simulink library "ifo"  (Simulink 8.2)
settings: Solver=ode45  StartTime=0.0  StopTime=10.0  RelTol=1e-3
undefined symbols (not defined in the file or in its folder): ENUM_EPSADASABREASON_NO_DRIVING_INTERRUPTION, ENUM_GEARPOSN_1ST, ENUM_GEARPOSN_2ND, ENUM_GEARPOSN_3RD, ENUM_GEARPOSN_4TH, ENUM_GEARPOSN_5TH, ENUM_GEARPOSN_6TH, ENUM_LFCSTATE_AUTOSTEERING, ENUM_LFCSTATE_DEGRADED, ENUM_SHIFTLEVER_D, ENUM_SHIFTLEVER_D2, ENUM_SHIFTLEVER_D3, FALSE, KAPP_VehicleWidth_m, KIFO_C1Max4Act_rad, KIFO_C2Max4Act_rat, KIFO_C2Max4Disable_rat, KIFO_C2Max4DisableThr_s, KIFO_DriverStrFightConfirmTime_s, KIFO_DriverStrFightResetTime_s, KIFO_DriverStrFightSetTime_s, KIFO_DriverStrFightThres_Nm, KIFO_DriverStrFightThresHys_Nm, KIFO_DriverStrSoftConfirmTime_s, KIFO_DriverStrSoftResetTime_s, KIFO_DriverStrSoftSetTime_s, KIFO_DriverStrSoftThres_Nm, KIFO_DriverStrStrongConfirmTime_s, KIFO_DriverStrStrongResetTime_s, KIFO_DriverStrStrongSetTime_s, KIFO_DriverStrStrongThres_Nm, KIFO_DriverStrStrongThresHys_Nm, KIFO_Lane4ActThr_s, KIFO_LaneWidthLowThr_m, KIFO_LaneWidthUpThr_m, KIFO_LFCVehSpdMaxLimition_kph, KIFO_LFCVehSpdMimLimition_kph, KIFO_LKAMaxActSpeed_kph, KIFO_LKAMaxDeactSpeed_kph, KIFO_LKAMinActSpeed_kph, KIFO_LKAMinDeactSpeed_kph, KIFO_TLCTriggerThrHysis_s, KIFO_TurnSignalSwOFFTime_s, MIFO_TLCThr4LKA_s, TRUE
libraries: hcu_lib x41, simulink x11, hmi x1, gaps x1, ttc x1, sft x1, veh x1
(part 2 of 2)

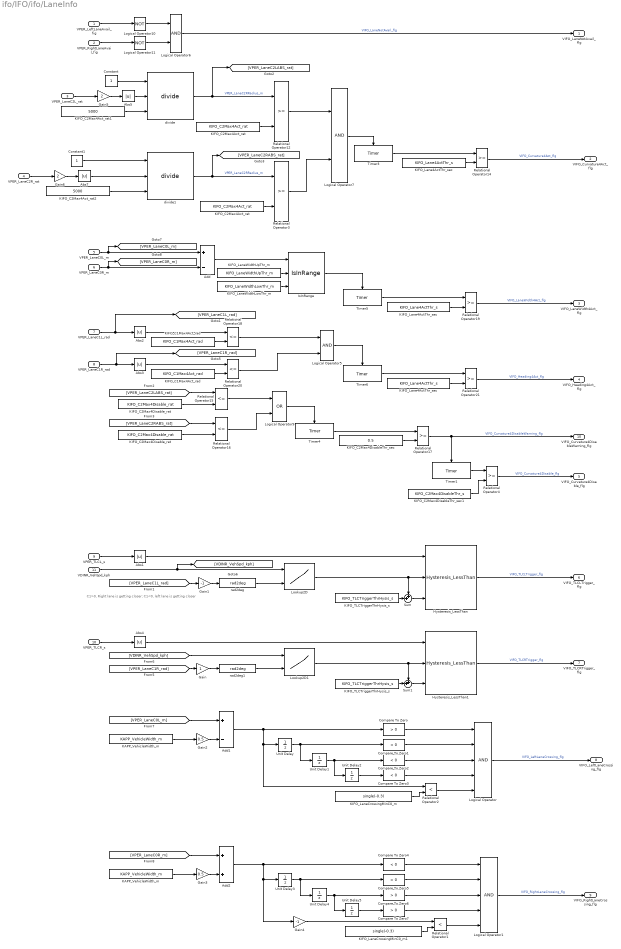
== system ifo/IFO/ifo/LaneInfo ==
  note: C1>0, Right lane is getting closer; C1<0, left lane is getting closer
  "VPER_LeftLaneAvail_fig " : Inport
  "VPER_RightLaneAvail_fig " : Inport  Port=2
  VPER_LaneC2L_rat : Inport  Port=3
  VPER_LaneC2R_rat : Inport  Port=4
  VPER_LaneC0L_m : Inport  Port=5
  VPER_LaneC0R_m : Inport  Port=6
  VPER_LaneC1L_rad : Inport  Port=7
  VPER_LaneC1R_rad : Inport  Port=8
  VPER_TLCL_s : Inport  Port=9
  VPER_TLCR_s : Inport  Port=10
  VDINR_VehSpd_kph : Inport  Port=11
  Abs{1..5,7} (6 alike) : Abs
  Add : Sum  Inputs=+-
  Add1 : Sum  Inputs=+-
  Add2 : Sum
  Compare To Zero{,5..7} (4 alike) : simulink/Logic and Bit Operations/Compare To Zero  relop=>  OutDataTypeStr=boolean
  Compare To Zero{1..4} (4 alike) : simulink/Logic and Bit Operations/Compare To Zero  relop=<  OutDataTypeStr=boolean
  Constant : Constant  OutDataTypeStr=single
  Constant1 : Constant  OutDataTypeStr=single
  Gain : Gain
  Gain1 : Gain  Gain=-1
  Gain2 : Gain  Gain=0.5
  Gain3 : Gain  Gain=0.5
  Gain4 : Gain  Gain=-1
  Gain5 : Gain  Gain=2
  Gain6 : Gain  Gain=2
  Hysteresis_LessThan : hcu_lib/Hysteresis_LessThan  SystemSampleTime=-1
  Hysteresis_LessThan1 : hcu_lib/Hysteresis_LessThan  SystemSampleTime=-1
  IsInRange : hcu_lib/IsInRange  SystemSampleTime=-1
  KAPP_VehicleWidth_m : Constant  Value=KAPP_VehicleWidth_m
  "KAPP_VehicleWidth_m " : Constant  Value=KAPP_VehicleWidth_m
  KIFO_C1Max4Act_rad : Constant  Value=KIFO_C1Max4Act_rad
  "KIFO_C1Max4Act_rad " : Constant  Value=KIFO_C1Max4Act_rad
  KIFO_C2Max4Act_rat : Constant  Value=KIFO_C2Max4Act_rat
  "KIFO_C2Max4Act_rat " : Constant  Value=KIFO_C2Max4Act_rat
  KIFO_C2Max4Act_rat1 : Constant  Value=5000  OutDataTypeStr=single
  KIFO_C2Max4Act_rat2 : Constant  Value=5000  OutDataTypeStr=single
  KIFO_C2Max4DisableThr_sec : Constant  Value=0.5
  KIFO_C2Max4DisableThr_sec1 : Constant  Value=KIFO_C2Max4DisableThr_s
  KIFO_C2Max4Disable_rat : Constant  Value=KIFO_C2Max4Disable_rat
  "KIFO_C2Max4Disable_rat " : Constant  Value=KIFO_C2Max4Disable_rat
  KIFO_Lane4ActThr_sec : Constant  Value=KIFO_Lane4ActThr_s
  "KIFO_Lane4ActThr_sec " : Constant  Value=KIFO_Lane4ActThr_s
  "KIFO_Lane4ActThr_sec   " : Constant  Value=KIFO_Lane4ActThr_s
  KIFO_LaneCrossingMinC0_m : Constant  Value=single(-0.3)
  KIFO_LaneCrossingMinC0_m1 : Constant  Value=single(-0.3)
  KIFO_LaneWidthLowThr_m : Constant  Value=KIFO_LaneWidthLowThr_m  OutDataTypeStr=single
  KIFO_LaneWidthUpThr_m : Constant  Value=KIFO_LaneWidthUpThr_m  OutDataTypeStr=single
  KIFO_TLCTriggerThrHysis_s : Constant  Value=KIFO_TLCTriggerThrHysis_s
  "KIFO_TLCTriggerThrHysis_s " : Constant  Value=KIFO_TLCTriggerThrHysis_s
  Logical Operator : Logic  Inputs=5  AllPortsSameDT=off  OutDataTypeStr=boolean
  Logical Operator1 : Logic  Inputs=5  AllPortsSameDT=off  OutDataTypeStr=boolean
  Logical Operator10 : Logic  Operator=NOT  AllPortsSameDT=off  OutDataTypeStr=boolean
  Logical Operator11 : Logic  Operator=NOT  AllPortsSameDT=off  OutDataTypeStr=boolean
  Logical Operator5 : Logic  AllPortsSameDT=off  OutDataTypeStr=boolean
  Logical Operator6 : Logic  AllPortsSameDT=off  OutDataTypeStr=boolean
  Logical Operator7 : Logic  AllPortsSameDT=off  OutDataTypeStr=boolean
  Logical Operator9 : Logic  Operator=OR  AllPortsSameDT=off  OutDataTypeStr=boolean
  Lookup2D : Lookup2D  RowIndex=AIFO_TLCThrVehSpd_X_kph  ColumnIndex=AIFO_TLCThrHeading_Y_deg  Table=MIFO_TLCThr4LKA_s  LookUpMeth=Interpolation-Use End Values  OutDataTypeStr=single
      settings: AttributesFormatString=|
      | <row=%<RowIndex>>
      | <column=%<ColumnIndex>>
      | <table=%<Table>>
  Lookup2D1 : Lookup2D  RowIndex=AIFO_TLCThrVehSpd_X_kph  ColumnIndex=AIFO_TLCThrHeading_Y_deg  Table=MIFO_TLCThr4LKA_s  LookUpMeth=Interpolation-Use End Values  OutDataTypeStr=single
      settings: AttributesFormatString=|
      | <row=%<RowIndex>>
      | <column=%<ColumnIndex>>
      | <table=%<Table>>
  Relational Operator1 : RelationalOperator  Operator=<  OutDataTypeStr=boolean
  Relational Operator{3..4,12,14,17,19,21} (7 alike) : RelationalOperator  OutDataTypeStr=boolean
  Relational Operator{15..16,18,20} (4 alike) : RelationalOperator  Operator=<=  OutDataTypeStr=boolean
  Relational Operator2 : RelationalOperator  Operator=<  OutDataTypeStr=boolean
  Sum : Sum  Inputs=++|
  Sum1 : Sum  Inputs=++|
  Timer{1,3..6} (5 alike) : hcu_lib/Timer  SystemSampleTime=-1
  Unit Delay{,1..5} (6 alike) : UnitDelay  SampleTime=-1
  divide : hcu_lib/divide
  divide1 : hcu_lib/divide
  rad2deg : hcu_lib/rad2deg
  rad2deg1 : hcu_lib/rad2deg
  VIFO_LaneNotAvail_flg : Outport
  VIFO_Curvature4Act_flg : Outport  Port=2
  VIFO_LaneWidth4Act_flg : Outport  Port=3
  VIFO_Heading4Act_flg : Outport  Port=4
  VIFO_Curvature4Disable_flg : Outport  Port=5
  VIFO_TLCLTrigger_flg : Outport  Port=6
  VIFO_TLCRTrigger_flg : Outport  Port=7
  VIFO_LeftLaneCrossing_flg : Outport  Port=8
  VIFO_RightLaneCrossing_flg : Outport  Port=9
  VIFO_Curvature4DisableWarning_flg : Outport  Port=10
  wires:
  KIFO_C1Max4Act_rad/1 -> Relational Operator18/2
  Relational Operator21/1 -> VIFO_Heading4Act_flg/1  "VIFO_Heading4Act_flg"
  "KIFO_Lane4ActThr_sec   "/1 -> Relational Operator21/2
  Timer6/1 -> Relational Operator21/1
  Logical Operator5/1 -> Timer6/Enable
  Relational Operator20/1 -> Logical Operator5/2
  Relational Operator18/1 -> Logical Operator5/1
  "KIFO_C1Max4Act_rad "/1 -> Relational Operator20/2
  VPER_LaneC1R_rad/1 -> [VPER_LaneC1R_rad], Abs3/1
  VPER_LaneC1L_rad/1 -> [VPER_LaneC1L_rad], Abs2/1
  Add/1 -> IsInRange/1
  Relational Operator19/1 -> VIFO_LaneWidth4Act_flg/1  "VIFO_LaneWidth4Act_flg"
  VPER_LaneC0R_m/1 -> [VPER_LaneC0R_m], Add/2
  "KIFO_Lane4ActThr_sec "/1 -> Relational Operator19/2
  Timer5/1 -> Relational Operator19/1
  VPER_LaneC0L_m/1 -> [VPER_LaneC0L_m], Add/1
  Relational Operator4/1 -> VIFO_Curvature4Disable_flg/1  "VIFO_Curvature4Disable_flg"
  Logical Operator6/1 -> VIFO_LaneNotAvail_flg/1  "VIFO_LaneNotAvail_flg"
  KIFO_C2Max4DisableThr_sec/1 -> Relational Operator17/2
  Timer4/1 -> Relational Operator17/1
  Logical Operator9/1 -> Timer4/Enable
  Relational Operator16/1 -> Logical Operator9/2
  Relational Operator15/1 -> Logical Operator9/1
  "KIFO_C2Max4Disable_rat "/1 -> Relational Operator16/2
  KIFO_C2Max4Disable_rat/1 -> Relational Operator15/2
  KIFO_C2Max4Act_rat/1 -> Relational Operator12/2
  Relational Operator14/1 -> VIFO_Curvature4Act_flg/1  "VIFO_Curvature4Act_flg"
  KIFO_Lane4ActThr_sec/1 -> Relational Operator14/2
  Timer3/1 -> Relational Operator14/1
  Logical Operator7/1 -> Timer3/Enable
  Relational Operator12/1 -> Logical Operator7/1
  "KIFO_C2Max4Act_rat "/1 -> Relational Operator3/2
  VPER_LaneC2L_rat/1 -> Gain5/1
  KIFO_LaneWidthUpThr_m/1 -> IsInRange/2
  KIFO_LaneWidthLowThr_m/1 -> IsInRange/3
  IsInRange/1 -> Timer5/Enable
  VPER_TLCL_s/1 -> Abs1/1
  VPER_TLCR_s/1 -> Abs4/1
  "VPER_RightLaneAvail_fig "/1 -> Logical Operator11/1
  "VPER_LeftLaneAvail_fig "/1 -> Logical Operator10/1
  Logical Operator10/1 -> Logical Operator6/1
  Logical Operator11/1 -> Logical Operator6/2
  [VPER_LaneC2LABS_rat] -> Relational Operator15/1
  [VPER_LaneC2RABS_rat] -> Relational Operator16/1
  Abs1/1 -> Hysteresis_LessThan/1
  Lookup2D/1 -> Sum/1, Hysteresis_LessThan/2
  Sum/1 -> Hysteresis_LessThan/3
  KIFO_TLCTriggerThrHysis_s/1 -> Sum/2
  Hysteresis_LessThan/1 -> VIFO_TLCLTrigger_flg/1  "VIFO_TLCLTrigger_flg"
  Lookup2D1/1 -> Hysteresis_LessThan1/2, Sum1/1
  Sum1/1 -> Hysteresis_LessThan1/3
  "KIFO_TLCTriggerThrHysis_s "/1 -> Sum1/2
  Abs4/1 -> Hysteresis_LessThan1/1
  Hysteresis_LessThan1/1 -> VIFO_TLCRTrigger_flg/1  "VIFO_TLCRTrigger_flg"
  Abs2/1 -> Relational Operator18/1
  Abs3/1 -> Relational Operator20/1
  [VPER_LaneC1L_rad] -> Gain1/1
  [VPER_LaneC1R_rad] -> Gain/1
  Gain/1 -> rad2deg1/1
  rad2deg/1 -> Lookup2D/2
  rad2deg1/1 -> Lookup2D1/2
  VDINR_VehSpd_kph/1 -> [VDINR_VehSpd_kph], Lookup2D/1
  [VDINR_VehSpd_kph] -> Lookup2D1/1
  Gain1/1 -> rad2deg/1
  Unit Delay/1 -> Unit Delay1/1, Compare To Zero1/1
  Compare To Zero/1 -> Logical Operator/1
  Compare To Zero1/1 -> Logical Operator/2
  Unit Delay1/1 -> Unit Delay2/1, Compare To Zero2/1
  Unit Delay2/1 -> Compare To Zero3/1
  Compare To Zero2/1 -> Logical Operator/3
  Compare To Zero3/1 -> Logical Operator/4
  Logical Operator/1 -> VIFO_LeftLaneCrossing_flg/1  "VIFO_LeftLaneCrossing_flg"
  Unit Delay3/1 -> Compare To Zero5/1, Unit Delay4/1
  Unit Delay4/1 -> Compare To Zero6/1, Unit Delay5/1
  Unit Delay5/1 -> Compare To Zero7/1
  KAPP_VehicleWidth_m/1 -> Gain2/1
  [VPER_LaneC0L_m] -> Add1/1
  Gain2/1 -> Add1/2
  "KAPP_VehicleWidth_m "/1 -> Gain3/1
  Gain3/1 -> Add2/2
  [VPER_LaneC0R_m] -> Add2/1
  Add1/1 -> Relational Operator2/1, Unit Delay/1, Compare To Zero/1
  KIFO_LaneCrossingMinC0_m/1 -> Relational Operator2/2
  Add2/1 -> Compare To Zero4/1, Gain4/1, Unit Delay3/1
  KIFO_LaneCrossingMinC0_m1/1 -> Relational Operator1/2
  Gain4/1 -> Relational Operator1/1
  Abs5/1 -> divide/2
  Constant/1 -> divide/1
  Gain5/1 -> Abs5/1
  Constant1/1 -> divide1/1
  VPER_LaneC2R_rat/1 -> Gain6/1
  Gain6/1 -> Abs7/1
  Abs7/1 -> divide1/2
  divide1/1 -> Relational Operator3/1, [VPER_LaneC2RABS_rat]  "VPER_LaneC2RRadius_m"
  Relational Operator3/1 -> Logical Operator7/2
  divide/1 -> [VPER_LaneC2LABS_rat], Relational Operator12/1  "VPER_LaneC2RRadius_m"
  KIFO_C2Max4Act_rat1/1 -> divide/3
  KIFO_C2Max4Act_rat2/1 -> divide1/3
  Relational Operator17/1 -> VIFO_Curvature4DisableWarning_flg/1, Timer1/Enable  "VIFO_Curvature4DisableWarning_flg"
  Timer1/1 -> Relational Operator4/1
  KIFO_C2Max4DisableThr_sec1/1 -> Relational Operator4/2
  Relational Operator2/1 -> Logical Operator/5
  Compare To Zero7/1 -> Logical Operator1/4
  Compare To Zero5/1 -> Logical Operator1/2
  Compare To Zero6/1 -> Logical Operator1/3
  Compare To Zero4/1 -> Logical Operator1/1
  Relational Operator1/1 -> Logical Operator1/5
  Logical Operator1/1 -> VIFO_RightLaneCrossing_flg/1  "VIFO_RightLaneCrossing_flg"

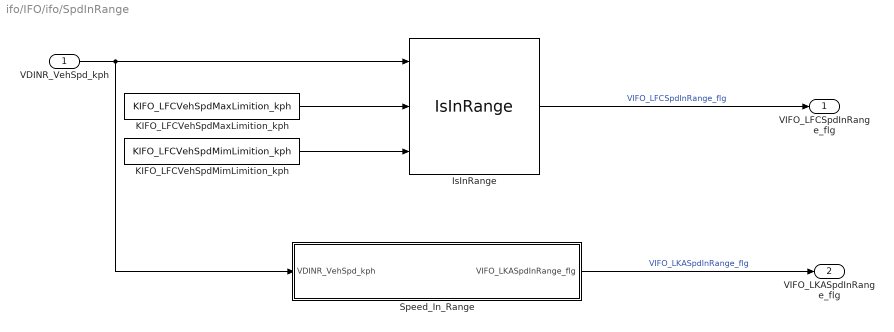
== system ifo/IFO/ifo/SpdInRange ==
  "VDINR_VehSpd_kph " : Inport
  IsInRange : hcu_lib/IsInRange  SystemSampleTime=-1
  KIFO_LFCVehSpdMaxLimition_kph : Constant  Value=KIFO_LFCVehSpdMaxLimition_kph
  KIFO_LFCVehSpdMimLimition_kph : Constant  Value=KIFO_LFCVehSpdMimLimition_kph
  Speed_In_Range : Subsystem
  VIFO_LFCSpdInRange_flg : Outport
  VIFO_LKASpdInRange_flg : Outport  Port=2
  wires:
  "VDINR_VehSpd_kph "/1 -> Speed_In_Range/1("VDINR_VehSpd_kph "), IsInRange/1
  KIFO_LFCVehSpdMaxLimition_kph/1 -> IsInRange/2
  KIFO_LFCVehSpdMimLimition_kph/1 -> IsInRange/3
  IsInRange/1 -> VIFO_LFCSpdInRange_flg/1  "VIFO_LFCSpdInRange_flg"
  Speed_In_Range/1(VIFO_LKASpdInRange_flg) -> VIFO_LKASpdInRange_flg/1  "VIFO_LKASpdInRange_flg"

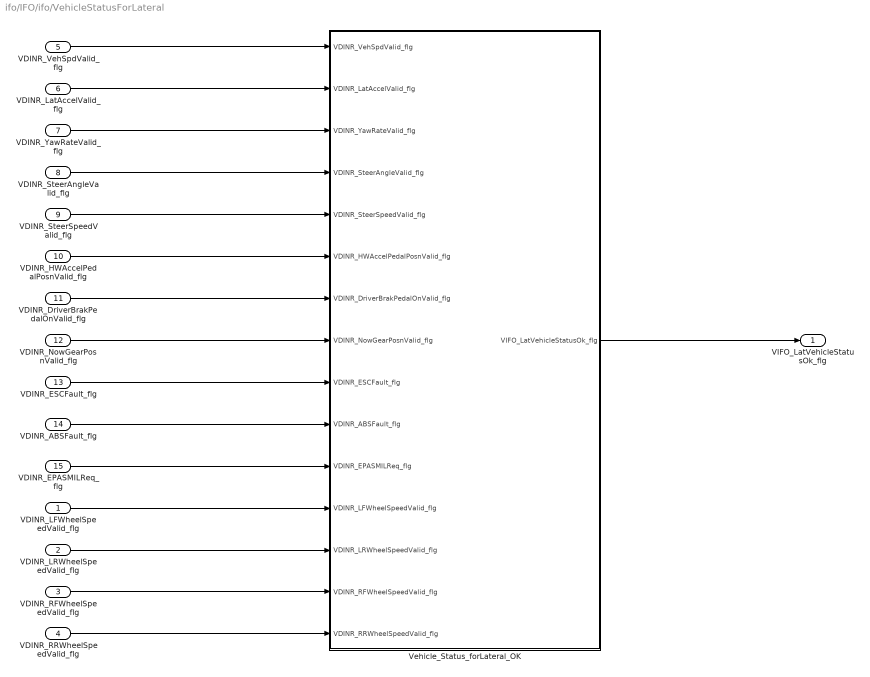
== system ifo/IFO/ifo/VehicleStatusForLateral ==
  VDINR_LFWheelSpeedValid_flg : Inport
  VDINR_LRWheelSpeedValid_flg : Inport  Port=2
  VDINR_RFWheelSpeedValid_flg : Inport  Port=3
  VDINR_RRWheelSpeedValid_flg : Inport  Port=4
  VDINR_VehSpdValid_flg : Inport  Port=5
  VDINR_LatAccelValid_flg : Inport  Port=6
  VDINR_YawRateValid_flg : Inport  Port=7
  VDINR_SteerAngleValid_flg : Inport  Port=8
  VDINR_SteerSpeedValid_flg : Inport  Port=9
  VDINR_HWAccelPedalPosnValid_flg : Inport  Port=10
  VDINR_DriverBrakPedalOnValid_flg : Inport  Port=11
  VDINR_NowGearPosnValid_flg : Inport  Port=12
  VDINR_ESCFault_flg : Inport  Port=13
  VDINR_ABSFault_flg : Inport  Port=14
  VDINR_EPASMILReq_flg : Inport  Port=15
  Vehicle_Status_forLateral_OK : Subsystem
  VIFO_LatVehicleStatusOk_flg : Outport
  wires:
  VDINR_EPASMILReq_flg/1 -> Vehicle_Status_forLateral_OK/11("VDINR_EPASMILReq_flg ")
  VDINR_ABSFault_flg/1 -> Vehicle_Status_forLateral_OK/10("VDINR_ABSFault_flg ")
  VDINR_ESCFault_flg/1 -> Vehicle_Status_forLateral_OK/9("VDINR_ESCFault_flg ")
  VDINR_NowGearPosnValid_flg/1 -> Vehicle_Status_forLateral_OK/8("VDINR_NowGearPosnValid_flg ")
  VDINR_DriverBrakPedalOnValid_flg/1 -> Vehicle_Status_forLateral_OK/7("VDINR_DriverBrakPedalOnValid_flg ")
  VDINR_HWAccelPedalPosnValid_flg/1 -> Vehicle_Status_forLateral_OK/6("VDINR_HWAccelPedalPosnValid_flg ")
  VDINR_SteerSpeedValid_flg/1 -> Vehicle_Status_forLateral_OK/5("VDINR_SteerSpeedValid_flg ")
  VDINR_SteerAngleValid_flg/1 -> Vehicle_Status_forLateral_OK/4("VDINR_SteerAngleValid_flg ")
  VDINR_YawRateValid_flg/1 -> Vehicle_Status_forLateral_OK/3("VDINR_YawRateValid_flg ")
  VDINR_VehSpdValid_flg/1 -> Vehicle_Status_forLateral_OK/1("VDINR_VehSpdValid_flg ")
  VDINR_LatAccelValid_flg/1 -> Vehicle_Status_forLateral_OK/2("VDINR_LatAccelValid_flg ")
  Vehicle_Status_forLateral_OK/1(VIFO_LatVehicleStatusOk_flg) -> VIFO_LatVehicleStatusOk_flg/1
  VDINR_LFWheelSpeedValid_flg/1 -> Vehicle_Status_forLateral_OK/12(VDINR_LFWheelSpeedValid_flg)
  VDINR_LRWheelSpeedValid_flg/1 -> Vehicle_Status_forLateral_OK/13(VDINR_LRWheelSpeedValid_flg)
  VDINR_RFWheelSpeedValid_flg/1 -> Vehicle_Status_forLateral_OK/14(VDINR_RFWheelSpeedValid_flg)
  VDINR_RRWheelSpeedValid_flg/1 -> Vehicle_Status_forLateral_OK/15(VDINR_RRWheelSpeedValid_flg)

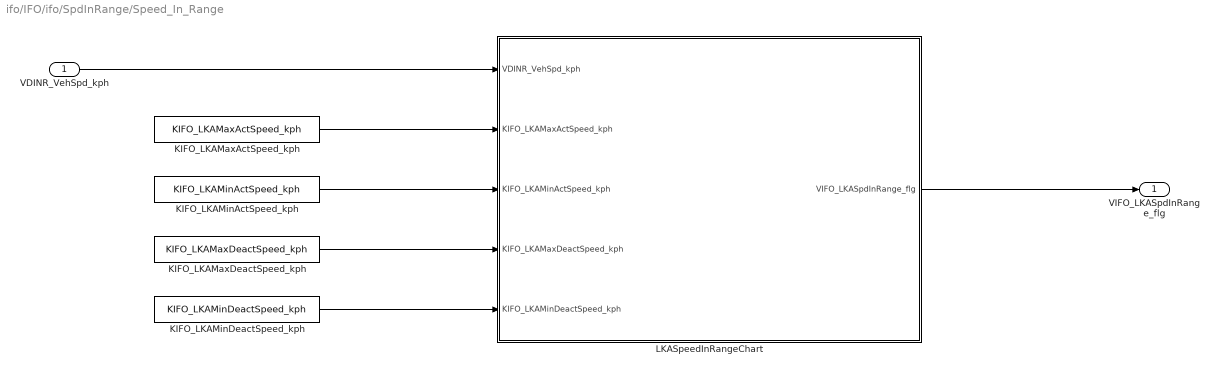
== system ifo/IFO/ifo/SpdInRange/Speed_In_Range ==
  "VDINR_VehSpd_kph " : Inport
  KIFO_LKAMaxActSpeed_kph : Constant  Value=KIFO_LKAMaxActSpeed_kph  OutDataTypeStr=single
  KIFO_LKAMaxDeactSpeed_kph : Constant  Value=KIFO_LKAMaxDeactSpeed_kph
  KIFO_LKAMinActSpeed_kph : Constant  Value=KIFO_LKAMinActSpeed_kph
  KIFO_LKAMinDeactSpeed_kph : Constant  Value=KIFO_LKAMinDeactSpeed_kph
  LKASpeedInRangeChart : Stateflow chart  TreatAsAtomicUnit=on
  VIFO_LKASpdInRange_flg : Outport
  wires:
  "VDINR_VehSpd_kph "/1 -> LKASpeedInRangeChart/1(VDINR_VehSpd_kph)
  LKASpeedInRangeChart/1(VIFO_LKASpdInRange_flg) -> VIFO_LKASpdInRange_flg/1
  KIFO_LKAMinActSpeed_kph/1 -> LKASpeedInRangeChart/3(KIFO_LKAMinActSpeed_kph)
  KIFO_LKAMaxActSpeed_kph/1 -> LKASpeedInRangeChart/2(KIFO_LKAMaxActSpeed_kph)
  KIFO_LKAMaxDeactSpeed_kph/1 -> LKASpeedInRangeChart/4(KIFO_LKAMaxDeactSpeed_kph)
  KIFO_LKAMinDeactSpeed_kph/1 -> LKASpeedInRangeChart/5(KIFO_LKAMinDeactSpeed_kph)

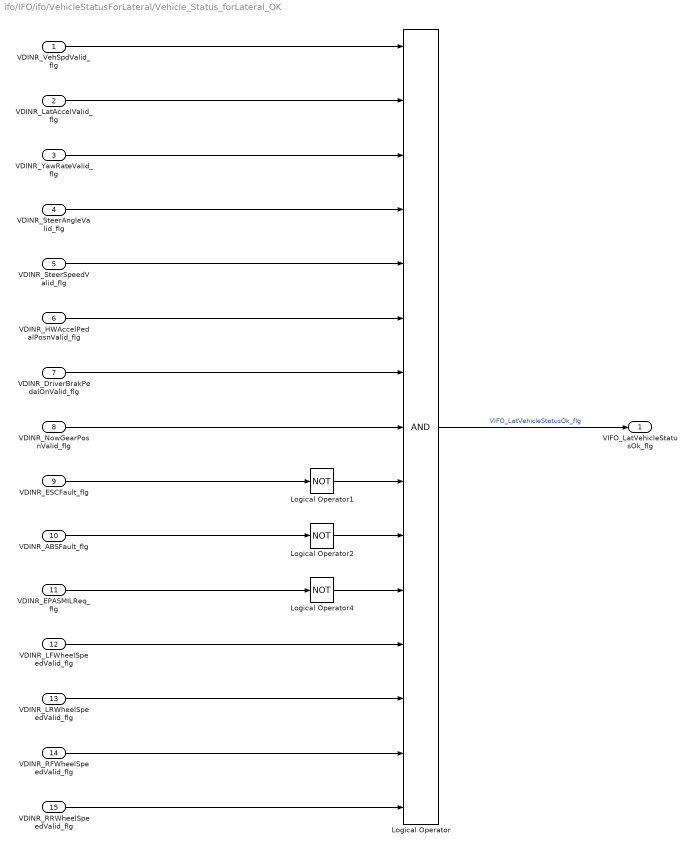
== system ifo/IFO/ifo/VehicleStatusForLateral/Vehicle_Status_forLateral_OK ==
  "VDINR_VehSpdValid_flg " : Inport
  "VDINR_LatAccelValid_flg " : Inport  Port=2
  "VDINR_YawRateValid_flg " : Inport  Port=3
  "VDINR_SteerAngleValid_flg " : Inport  Port=4
  "VDINR_SteerSpeedValid_flg " : Inport  Port=5
  "VDINR_HWAccelPedalPosnValid_flg " : Inport  Port=6
  "VDINR_DriverBrakPedalOnValid_flg " : Inport  Port=7
  "VDINR_NowGearPosnValid_flg " : Inport  Port=8
  "VDINR_ESCFault_flg " : Inport  Port=9
  "VDINR_ABSFault_flg " : Inport  Port=10
  "VDINR_EPASMILReq_flg " : Inport  Port=11
  VDINR_LFWheelSpeedValid_flg : Inport  Port=12
  VDINR_LRWheelSpeedValid_flg : Inport  Port=13
  VDINR_RFWheelSpeedValid_flg : Inport  Port=14
  VDINR_RRWheelSpeedValid_flg : Inport  Port=15
  Logical Operator : Logic  Inputs=15  AllPortsSameDT=off  OutDataTypeStr=boolean
  Logical Operator1 : Logic  Operator=NOT  AllPortsSameDT=off  OutDataTypeStr=boolean
  Logical Operator2 : Logic  Operator=NOT  AllPortsSameDT=off  OutDataTypeStr=boolean
  Logical Operator4 : Logic  Operator=NOT  AllPortsSameDT=off  OutDataTypeStr=boolean
  VIFO_LatVehicleStatusOk_flg : Outport
  wires:
  "VDINR_VehSpdValid_flg "/1 -> Logical Operator/1
  Logical Operator/1 -> VIFO_LatVehicleStatusOk_flg/1  "VIFO_LatVehicleStatusOk_flg"
  "VDINR_ESCFault_flg "/1 -> Logical Operator1/1
  "VDINR_ABSFault_flg "/1 -> Logical Operator2/1
  "VDINR_EPASMILReq_flg "/1 -> Logical Operator4/1
  "VDINR_LatAccelValid_flg "/1 -> Logical Operator/2
  "VDINR_SteerAngleValid_flg "/1 -> Logical Operator/4
  "VDINR_DriverBrakPedalOnValid_flg "/1 -> Logical Operator/7
  "VDINR_NowGearPosnValid_flg "/1 -> Logical Operator/8
  "VDINR_YawRateValid_flg "/1 -> Logical Operator/3
  "VDINR_HWAccelPedalPosnValid_flg "/1 -> Logical Operator/6
  "VDINR_SteerSpeedValid_flg "/1 -> Logical Operator/5
  Logical Operator2/1 -> Logical Operator/10
  Logical Operator1/1 -> Logical Operator/9
  Logical Operator4/1 -> Logical Operator/11
  VDINR_RRWheelSpeedValid_flg/1 -> Logical Operator/15
  VDINR_RFWheelSpeedValid_flg/1 -> Logical Operator/14
  VDINR_LRWheelSpeedValid_flg/1 -> Logical Operator/13
  VDINR_LFWheelSpeedValid_flg/1 -> Logical Operator/12

== stateflow chart IFO/ifo/SpdInRange/Speed_In_Range/LKASpeedInRangeChart ==
  state SPEED_OUT_OF_RANGE
    en:
    VIFO_LKASpdInRange_flg=FALSE;
  state SPEED_IN_RANGE
    en:
    VIFO_LKASpdInRange_flg = TRUE;
  (default) -> SPEED_OUT_OF_RANGE
  SPEED_OUT_OF_RANGE -> SPEED_IN_RANGE : [(VDINR_VehSpd_kph>KIFO_LKAMinActSpeed_kph)&&...
      | (VDINR_VehSpd_kph<KIFO_LKAMaxActSpeed_kph)]
  SPEED_IN_RANGE -> SPEED_OUT_OF_RANGE : [(VDINR_VehSpd_kph<KIFO_LKAMinDeactSpeed_kph)||...
      | (VDINR_VehSpd_kph>KIFO_LKAMaxDeactSpeed_kph)]
  data: VDINR_VehSpd_kph input single; VIFO_LKASpdInRange_flg output boolean; FALSE parameter boolean; TRUE parameter boolean; KIFO_LKAMaxActSpeed_kph input single; KIFO_LKAMinActSpeed_kph input single; KIFO_LKAMaxDeactSpeed_kph input single; KIFO_LKAMinDeactSpeed_kph input single
